simulink model "nj"  (R2017a)
settings: Solver=VariableStepAuto  StartTime=0.0  StopTime=20.0  RelTol=1e-3
settings Model: Creator=mohammadst99  LastModifiedBy=mohammadst99

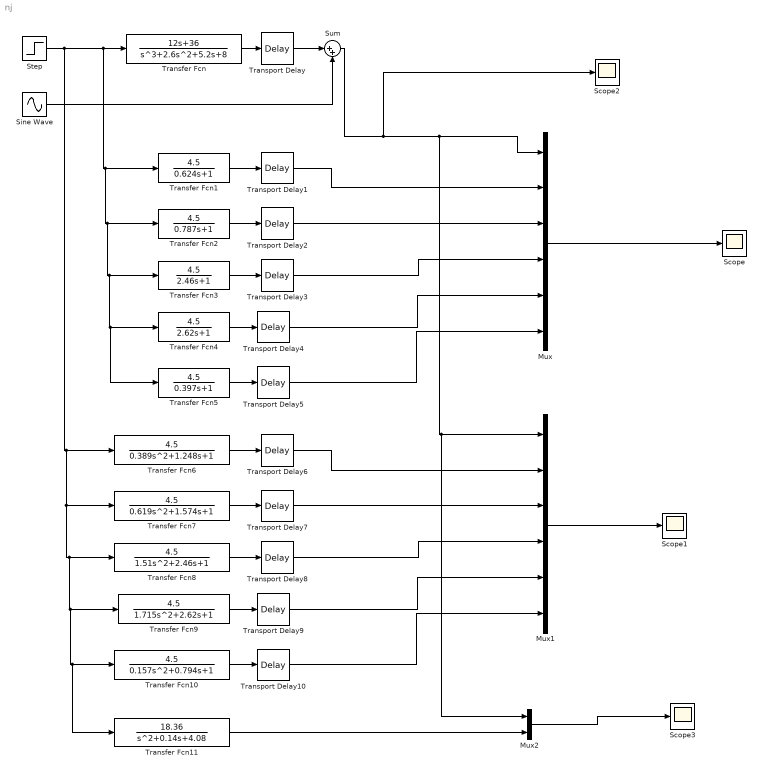
== system nj ==
  Mux : Mux  Inputs=6
  Mux1 : Mux  Inputs=6
  Mux2 : Mux  Inputs=2
  Scope{,1..3} (4 alike) : Scope
  Sine Wave : Sin  Amplitude=0.03  Frequency=40  SampleTime=0
  Step : Step  Time=0  SampleTime=0
  Sum : Sum  Inputs=|++
  Transfer Fcn : TransferFcn  Numerator=[12 36]  Denominator=[1 2.6 5.2 8]
  Transfer Fcn1 : TransferFcn  Numerator=[4.5]  Denominator=[0.624 1]
  Transfer Fcn10 : TransferFcn  Numerator=[4.5]  Denominator=[0.157 0.794 1]
  Transfer Fcn11 : TransferFcn  Numerator=[18.36]  Denominator="[1 0.14  4.08]"
  Transfer Fcn2 : TransferFcn  Numerator=[4.5]  Denominator=[0.787 1]
  Transfer Fcn3 : TransferFcn  Numerator=[4.5]  Denominator=[2.46 1]
  Transfer Fcn4 : TransferFcn  Numerator=[4.5]  Denominator=[2.62 1]
  Transfer Fcn5 : TransferFcn  Numerator=[4.5]  Denominator=[0.397 1]
  Transfer Fcn6 : TransferFcn  Numerator=[4.5]  Denominator=[0.389 1.248 1]
  Transfer Fcn7 : TransferFcn  Numerator=[4.5]  Denominator=[0.619 1.574 1]
  Transfer Fcn8 : TransferFcn  Numerator=[4.5]  Denominator=[1.51 2.46 1]
  Transfer Fcn9 : TransferFcn  Numerator=[4.5]  Denominator=[1.715 2.62 1]
  Transport Delay : TransportDelay  DelayTime=0.4
  Transport Delay{1,3,6,8} (4 alike) : TransportDelay  DelayTime=0.761
  Transport Delay10 : TransportDelay  DelayTime=0.732
  Transport Delay{2,4,7,9} (4 alike) : TransportDelay  DelayTime=0.598
  Transport Delay5 : TransportDelay  DelayTime=0.732
  wires:
  Transport Delay/1 -> Sum/1
  Step/1 -> Transfer Fcn11/1, Transfer Fcn10/1, Transfer Fcn9/1, Transfer Fcn8/1, Transfer Fcn7/1, Transfer Fcn6/1, Transfer Fcn5/1, Transfer Fcn4/1, Transfer Fcn3/1, Transfer Fcn2/1, Transfer Fcn1/1, Transfer Fcn/1
  Sine Wave/1 -> Sum/2
  Transfer Fcn/1 -> Transport Delay/1
  Sum/1 -> Scope2/1, Mux2/1, Mux1/1, Mux/1
  Mux/1 -> Scope/1
  Transfer Fcn5/1 -> Transport Delay5/1
  Transfer Fcn4/1 -> Transport Delay4/1
  Transfer Fcn3/1 -> Transport Delay3/1
  Transfer Fcn2/1 -> Transport Delay2/1
  Transfer Fcn1/1 -> Transport Delay1/1
  Transport Delay1/1 -> Mux/2
  Transport Delay2/1 -> Mux/3
  Transport Delay3/1 -> Mux/4
  Transport Delay4/1 -> Mux/5
  Transport Delay5/1 -> Mux/6
  Transfer Fcn9/1 -> Transport Delay9/1
  Transport Delay9/1 -> Mux1/5
  Transfer Fcn8/1 -> Transport Delay8/1
  Transfer Fcn10/1 -> Transport Delay10/1
  Transport Delay6/1 -> Mux1/2
  Transfer Fcn7/1 -> Transport Delay7/1
  Transfer Fcn6/1 -> Transport Delay6/1
  Transport Delay7/1 -> Mux1/3
  Transport Delay8/1 -> Mux1/4
  Transport Delay10/1 -> Mux1/6
  Mux1/1 -> Scope1/1
  Mux2/1 -> Scope3/1
  Transfer Fcn11/1 -> Mux2/2
